simulink model "rrc_v_rect_bw"  (Simulink 6.6)
settings: Solver=ode45  StartTime=0.0  StopTime=0.5  RelTol=1e-3
PreLoadFcn:
  | rrc_weights
  | filter_weights
StopFcn:
  | figure(15)
  | 
  | subplot(2,1,1)
  | plot(i_rect,'b');
  | xlabel('Samples');
  | ylabel('Amplitude');
  | legend('Rectangular Shaped',1);
  | axis([0 10000 -1.5 1.5]);
  | 
  | subplot(2,1,2)
  | plot(i_rrc,'k');
  | xlabel('Samples');
  | ylabel('Amplitude');
  | legend('RRC Shaped',1);
  | axis([0 10000 -1.5 1.5]);
  | 
  | doFFTplot(153.6e+3, i_rrc_if,'Modulated (I, RRC)',1,16);
  | axis([0 7.68e4 -40 80]);
  | doFFTplot(153.6e+3, i_rect_if,'Modulated (I, Rectangular)',1,17);
  | axis([0 7.68e4 -40 80]);
libraries: dsparch4 x2, dspsigops x1
settings Model: Creator=lcrockett  LastModifiedBy=lcrockett

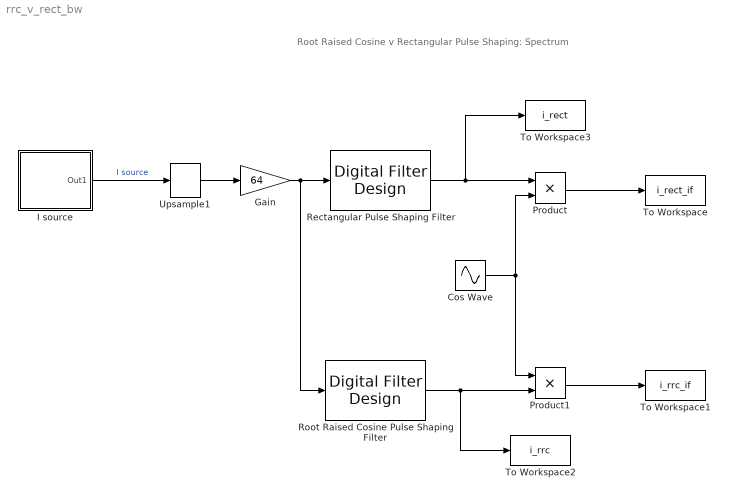
== system rrc_v_rect_bw ==
  note: Root Raised Cosine v Rectangular Pulse Shaping: Spectrum
  Cos Wave : Sin  Frequency=(38.4e+3)*2*pi  Phase=pi/2  SampleTime=1/153.6e+3
  Gain : Gain  Gain=64
  I source : Subsystem
  Product : Product  RndMeth=Zero
  Product1 : Product  RndMeth=Zero
  Rectangular Pulse Shaping Filter : dsparch4/Digital Filter Design  SystemSampleTime=-1  mwdsp_browser_bugfix_var=off
  Root Raised Cosine Pulse Shaping Filter : dsparch4/Digital Filter Design  SystemSampleTime=-1  mwdsp_browser_bugfix_var=off
  To Workspace : ToWorkspace  VariableName=i_rect_if  SampleTime=-1  SaveFormat=Array
  To Workspace1 : ToWorkspace  VariableName=i_rrc_if  SampleTime=-1  SaveFormat=Array
  To Workspace2 : ToWorkspace  VariableName=i_rrc  SampleTime=-1  SaveFormat=Array
  To Workspace3 : ToWorkspace  VariableName=i_rect  SampleTime=-1  SaveFormat=Array
  Upsample1 : dspsigops/Upsample  N=64  phase=0  ic=0  mode=Maintain input frame size
  wires:
  Rectangular Pulse Shaping Filter/1 -> Product/1, To Workspace3/1
  Product/1 -> To Workspace/1
  I source/1(Out1) -> Upsample1/1  "I source"
  Upsample1/1 -> Gain/1
  Cos Wave/1 -> Product/2, Product1/1
  Gain/1 -> Root Raised Cosine Pulse Shaping Filter/1, Rectangular Pulse Shaping Filter/1
  Root Raised Cosine Pulse Shaping Filter/1 -> To Workspace2/1, Product1/2
  Product1/1 -> To Workspace1/1

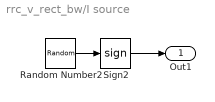
== system rrc_v_rect_bw/I source ==
  Random Number2 : RandomNumber  Seed=777  SampleTime=1/2400
  Sign2 : Signum
  Out1 : Outport
  wires:
  Random Number2/1 -> Sign2/1
  Sign2/1 -> Out1/1
